simulink model "AOO"  (R2022b)
settings: Solver=FixedStepAuto  StartTime=0.0  StopTime=10.0  FixedStep=1e-3  RelTol=1e-3  EnableMultiTasking=on
undefined symbols (not defined in the file): D10, D11, D12, D2, D4, D5, D7, D8, D9, PTA0, PTA2, PTB23, PTB9, PTC3, PTC4, PTD0, PTD2, PTD3
libraries: frdmk64flib x9
settings Model: ExtModeTrigDuration=5  Creator=16475  LastModifiedBy=kaano
settings OptimizationCC: EnhancedBackFolding=on  PassReuseOutputArgsAs=Individual arguments  ZeroExternalMemoryAtStartup=off  ZeroInternalMemoryAtStartup=off  MaxStackSize=64  OptimizeBlockOrder=speed  DifferentSizesBufferReuse=on  OptimizationCustomize=off  EfficientTunableParamExpr=on
settings DebuggingCC: ParameterTunabilityLossMsg=error
settings HardwareCC: ProdBitPerPointer=32  ProdBitPerSizeT=32  ProdBitPerPtrDiffT=32  ProdLargestAtomicInteger=Long  ProdLargestAtomicFloat=Double  ProdWordSize=32  ProdHWDeviceType=ARM Compatible->ARM Cortex
settings SFSimCC: MATLABDynamicMemAlloc=off
settings RTWCC: Description=Embedded Coder  SystemTargetFile=ert.tlc  HardwareBoard=NXP FRDM-K64F  TLCOptions="-aInlineSetEventsForThisBaseRateFcn=TLC_FALSE -aSuppressMultiTaskScheduler=TLC_FALSE  -aRateBasedStepFcn=0"  TemplateMakefile=ert_default_tmf  Toolchain=GNU Tools for ARM Embedded Processors
settings CodeAppCC: ForceParamTrailComments=on  IgnoreCustomStorageClasses=off  OperatorAnnotations=on  SimulinkDataObjDesc=on  SFDataObjDesc=on  InsertBlockDesc=on
settings ERTTargetCC: ExtModeTransport=4  ExtModeMexFile=sendToCommService

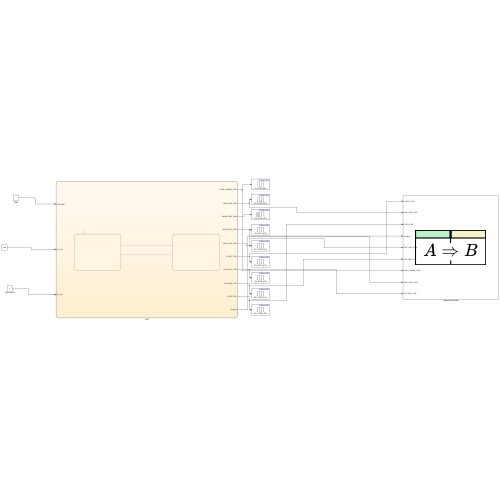
[thumbnail: Simulink's stored preview of the top-level diagram]
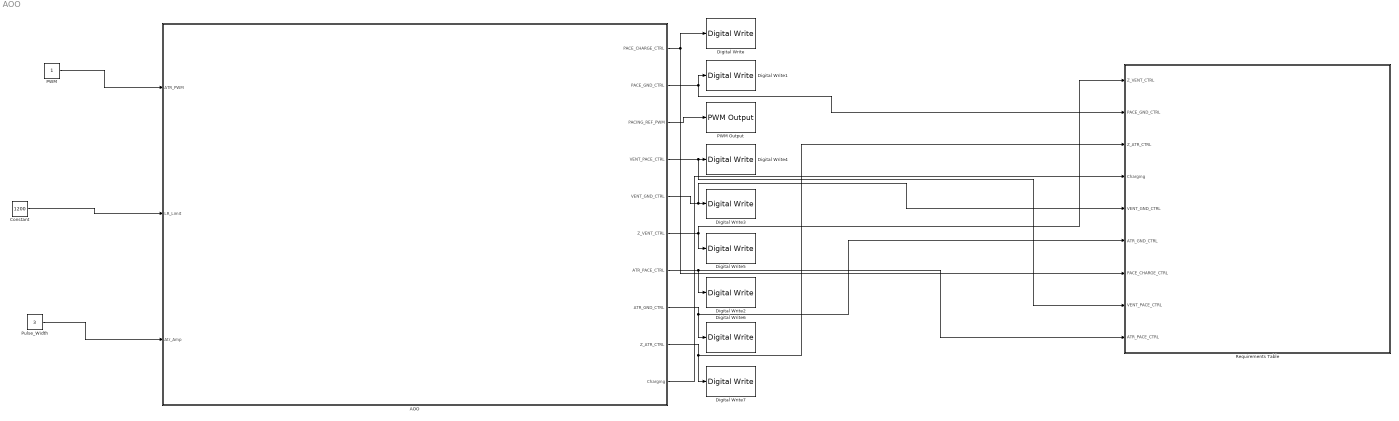
== system AOO ==
  AOO : Stateflow chart  TreatAsAtomicUnit=on
      settings: PortSchema="{\"entries\":[{\"content\":{\"sides\":[{\"content\":{\"connectorIds\":[\"In1\",\"In2\",\"In3\"]},\"type\":\"ConnectorPlacement.EquallySpacedRectSide\",\"uuid\":\"a3e94f58-3093-42a5-91db-f56c9d127bee\"},{\"content\":{\"connectorIds\":[\"Out1\",\"Out2\",\"Out3\",\"Out5\",\"Out4\",\"Out7\",\"Out6\",\"Out8\",\"Out9\",\"Out10\"],\"side\":\"RIGHT\"},\"type\":\"ConnectorPlacement.EquallySpacedRectSide\",\"uuid\":\"289ad049-9840-4721-af22-1385d5696f7c\"},{\"content\":{\"connectorIds\":[],\"side\":\"TOP\"},\"type\":\"ConnectorPlacement.EquallySpacedRectSide\",\"uuid\":\"4602f2ad-cb91-4c7a-9db6-6571445db01f\"}]},\"type\":\"ConnectorPlacement.EquallySpacedConnector\",\"uuid\":\"bfd50937-4990-4c1b-ba87-ff4dc7d3240f\"}],\"packageUris\":[\"http://schema.mathworks.com/mf0/Connector/R2020b\"],\"version\":\"1.0\"}"
  Constant : Constant  Value=1200
  Digital Write : frdmk64flib/Digital Write  Whichpin=PTB9 (D2)
  Digital Write1 : frdmk64flib/Digital Write  Whichpin=PTD0 (D10)
  Digital Write2 : frdmk64flib/Digital Write  Whichpin=PTA0 (D8)
  Digital Write3 : frdmk64flib/Digital Write  Whichpin=PTD3 (D12)
  Digital Write4 : frdmk64flib/Digital Write  Whichpin=PTC4 (D9)
  Digital Write5 : frdmk64flib/Digital Write  Whichpin=PTC3 (D7)
  Digital Write6 : frdmk64flib/Digital Write  Whichpin=PTD2 (D11)
  Digital Write7 : frdmk64flib/Digital Write  Whichpin=PTB23 (D4)
  PWM : Constant
  PWM Output : frdmk64flib/PWM Output  Whichpin=PTA2 (D5)  InitialFrequency=2000  InitialDutyCycle=0
  Pulse_Width : Constant  Value=3
  Requirements Table : Requirements Table  TreatAsAtomicUnit=on
  wires:
  AOO/8(ATR_GND_CTRL) -> Requirements Table/6(ATR_GND_CTRL), Digital Write6/1
  AOO/7(Z_VENT_CTRL) -> Digital Write5/1, Requirements Table/1(Z_VENT_CTRL)
  AOO/4(VENT_GND_CTRL) -> Requirements Table/5(VENT_GND_CTRL), Digital Write3/1
  AOO/2(PACE_GND_CTRL) -> Digital Write1/1, Requirements Table/2(PACE_GND_CTRL)
  AOO/1(PACE_CHARGE_CTRL) -> Requirements Table/7(PACE_CHARGE_CTRL), Digital Write/1
  AOO/3(PACING_REF_PWM) -> PWM Output/1
  AOO/6(ATR_PACE_CTRL) -> Requirements Table/9(ATR_PACE_CTRL), Digital Write2/1
  AOO/9(Z_ATR_CTRL) -> Digital Write7/1, Requirements Table/3(Z_ATR_CTRL)
  AOO/5(VENT_PACE_CTRL) -> Requirements Table/8(VENT_PACE_CTRL), Digital Write4/1
  Pulse_Width/1 -> AOO/3(Atr_Amp)
  PWM/1 -> AOO/1(ATR_PWM)
  Constant/1 -> AOO/2(LR_Limit)
  AOO/10(Charging) -> Requirements Table/4(Charging)

== stateflow chart AOO/AOO ==
  state Charging
    entry:
    ATR_PACE_CTRL = false;
    VENT_PACE_CTRL = false;
    PACING_REF_PWM = ((Atr_Amp/5)*100);
    PACE_CHARGE_CTRL = true;
    PACE_GND_CTRL = true;
    Z_ATR_CTRL = false;
    Z_VENT_CTRL = false;
    ATR_GND_CTRL = true;
    VENT_GND_CTRL = false;
    Charging = true;
  state Pacing
    entry:
    PACE_CHARGE_CTRL = false;
    PACE_GND_CTRL = true;
    ATR_PACE_CTRL = true;
    VENT_PACE_CTRL = false;
    Z_ATR_CTRL = false;
    Z_VENT_CTRL = false;
    ATR_GND_CTRL = false;
    VENT_GND_CTRL = false;
    Charging = false;
  (default) -> Charging
  Charging -> Pacing : [after(LR_Limit - ATR_PWM,msec)]
  Pacing -> Charging : [after(ATR_PWM,msec)]
  data: ATR_PWM input double; LR_Limit input double; PACE_CHARGE_CTRL output boolean; PACE_GND_CTRL output boolean; PACING_REF_PWM output double; VENT_GND_CTRL output boolean; VENT_PACE_CTRL output boolean; ATR_PACE_CTRL output boolean; Z_VENT_CTRL output boolean; Atr_Amp input double; ATR_GND_CTRL output boolean; Z_ATR_CTRL output boolean; Charging output

== stateflow chart AOO/Requirements Table ==
  (default) -> (junction 1073741979)
  (junction 1073741979) -> (junction 1073741980) : {
      | % SF_REQ_REV_07
      | }
  (junction 1073741980) -> (junction 1073741982) : {
      | % HEADER_ASSIGNMENTS
      |
      | }
  (junction 1073741982) -> (junction 1073741984) : {
      | % START_A_4
      | }
  (junction 1073741984) -> (junction 1073741986) : {
      | }
  (junction 1073741986) -> (junction 1073741988)
  (junction 1073741988) -> (junction 1073741990) : {
      | }
  (junction 1073741990) -> (junction 1073741992) : {
      | % END_A_4
      | }
  (junction 1073741992) -> (junction 1073741994) : {
      | % START_R_1
      | }
  (junction 1073741994) -> (junction 1073741996) : {
      | }
  (junction 1073741996) -> (junction 1073741998)
  (junction 1073741998) -> (junction 1073742000) [order 1] : [(((prev(Charging)) == (prev(Charging) == false)))]
  (junction 1073741998) -> (junction 1073742006) [order 2]
  (junction 1073742000) -> (junction 1073742002) : {
      | reqtable_postcondition((((VENT_PACE_CTRL) == (false))) && (((PACE_CHARGE_CTRL ) == (true))) && (((PACE_GND_CTRL ) == (true))) && (((Z_ATR_CTRL ) == (false))) && (((ATR_PACE_CTRL ) == (false))) && (((VENT_GND_CTRL ) == (false))) && (((Z_VENT_CTRL ) == (false))) && (((ATR_GND_CTRL ) == (true))) && (((Charging) == (true))), 'R:1');
      |
      |
      | }
  (junction 1073742002) -> (junction 1073742004) : {
      | }
  (junction 1073742004) -> (junction 1073742006)
  (junction 1073742006) -> (junction 1073742008)
  (junction 1073742008) -> (junction 1073742010) : {
      | % END_R_1
      | }
  (junction 1073742010) -> (junction 1073742012) : {
      | % START_R_7
      | }
  (junction 1073742012) -> (junction 1073742014) : {
      | }
  (junction 1073742014) -> (junction 1073742016)
  (junction 1073742016) -> (junction 1073742018) [order 1] : [(((prev(Charging)) == (prev(Charging) == true)))]
  (junction 1073742016) -> (junction 1073742024) [order 2]
  (junction 1073742018) -> (junction 1073742020) : {
      | reqtable_postcondition((((VENT_PACE_CTRL) == (false))) && (((PACE_CHARGE_CTRL ) == (false))) && (((PACE_GND_CTRL ) == (true))) && (((Z_ATR_CTRL ) == (false))) && (((ATR_PACE_CTRL ) == (true))) && (((VENT_GND_CTRL ) == (false))) && (((Z_VENT_CTRL ) == (false))) && (((ATR_GND_CTRL ) == (false))) && (((Charging) == (false))), 'R:2');
      |
      |
      | }
  (junction 1073742020) -> (junction 1073742022) : {
      | }
  (junction 1073742022) -> (junction 1073742024)
  (junction 1073742024) -> (junction 1073742026)
  (junction 1073742026) -> (junction 1073742028) : {
      | % END_R_7
      | }
  data: Z_VENT_CTRL input; PACE_GND_CTRL input; Z_ATR_CTRL input; Charging input; VENT_GND_CTRL input; ATR_GND_CTRL input; PACE_CHARGE_CTRL input; VENT_PACE_CTRL input; ATR_PACE_CTRL input
